simulink model "Monorail_Phase_Shifted_Full_Bridge_Converter"  (R2021b)
settings: Solver=ode1  StartTime=0.0  StopTime=4.00  FixedStep=1e-6  MaxStep=1e-4  RelTol=1e-3  EnableMultiTasking=on
InitFcn:
  | %Input
  | V_supply_max = 910;
  | V_supply_min = 490;
  | R_supply = 1e-06;
  | L_in = 0.5e-03;
  | C_in = 225e-06;
  | 
  | %Control
  | f_sw = 10e03;
  | V_dc_ref = 750;
  | V_dc_init = 450;
  | V_bat_ref = 24;
  | V_bat_init = 14;
  | t_softstart = 0.5;
  | Scale_factor_High = 1/790;
  | Scale_factor_Low = 1/26.26;
  | Kp = 0.5;
  | Ki = pi;
  | PI_max = 0.95;
  | PI_min = 0.05;
  | t_enable = 1e-03;
  | t_dead = 2e-06;
  | 
  | %HF_Transformer
  | P_txf = 50e03;
  | f_txf = 10e03;
  | V_pri_txf = 1e03;
  | V_sec_high_txf = 770;
  | V_sec_low_txf = 27;
  | 
  | %Output
  | L_filt = 1e-03;
  | C_filt = 225e-06;
  | R_load_750V = 750/40;
  | R_load_24V = 24/500;
libraries: spsDiodeLib x12, spsSeriesRLCBranchLib x10, spsIGBTDiodeLib x8, spsCurrentMeasurementLib x3, spsVoltageMeasurementLib x3, simulink x3, spsLinearTransformerLib x2, simulink_extras x2, slpidlib x1, spsControlledVoltageSourceLib x1, spspowerguiLib x1
settings Model: ModifiedByFormat=Sourjya_Mondal  Creator=Sourjya_Mondal  LastModifiedBy=Sourjya_Mondal
settings SolverCC: AlgebraicLoopSolver=TrustRegion
settings DataIOCC: ReturnWorkspaceOutputs=off
settings OptimizationCC: LifeSpan=inf
settings DebuggingCC: SFUnexpectedBacktrackingDiag=warning  SFNoUnconditionalDefaultTransitionDiag=warning  SFExecutionAtInitializationDiag=none  SFMachineParentedDataDiag=warning  ArithmeticOperatorsInVariantConditions=warning
settings SFSimCC: SimUseLocalCustomCode=off  CustomCodeUndefinedFunction=UseInterfaceOnly
settings RTWCC: RTWUseLocalCustomCode=off
settings CodeAppCC: StateflowObjectComments=on
settings GRTTargetCC: TargetLangStandard=C89/C90 (ANSI)
settings ConfigComp: CovMetricSettings=dw  CovSaveCumulativeToWorkspaceVar=on  CovSaveSingleToWorkspaceVar=on  CovExternalEMLEnable=off
settings SimscapeCC: SimscapeNormalizeSystem=off

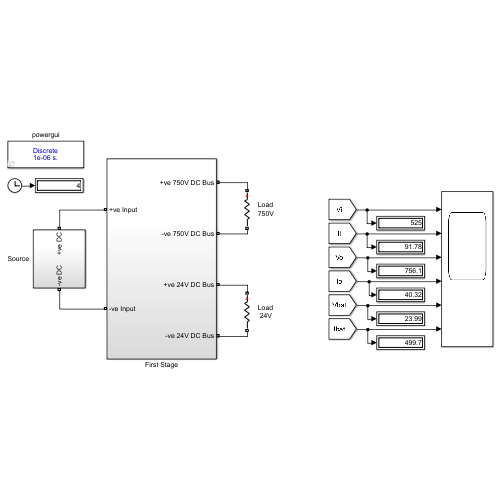
[thumbnail: Simulink's stored preview of the top-level diagram]
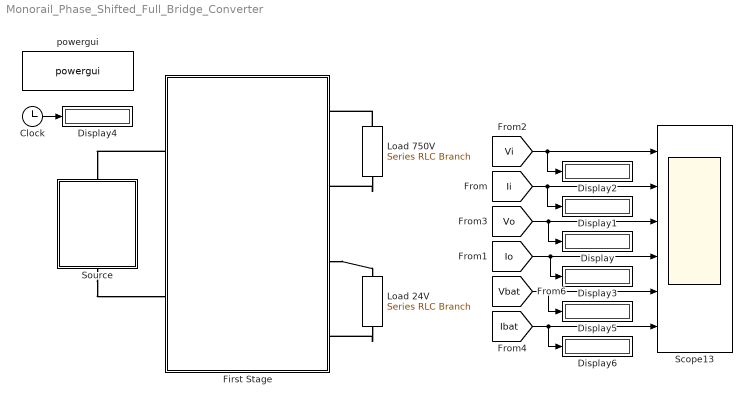
== system Monorail_Phase_Shifted_Full_Bridge_Converter ==
  Clock : Clock
  Display{,1..6} (7 alike) : Display
  First Stage : Subsystem
  Load 24V : spsSeriesRLCBranchLib/Series RLC Branch  LConnTagsString=__new0  RConnTagsString=__new0  BranchType=R  Resistance=R_load_24V  Inductance=1e-3  SetiL0=off  InitialCurrent=0  Capacitance=1e-6  Setx0=off  InitialVoltage=0  Measurements=None
  Load 750V : spsSeriesRLCBranchLib/Series RLC Branch  LConnTagsString=__new0  RConnTagsString=__new0  BranchType=R  Resistance=R_load_750V  Inductance=1e-3  SetiL0=off  InitialCurrent=0  Capacitance=1e-6  Setx0=off  InitialVoltage=0  Measurements=None
  Scope13 : Scope  NumInputPorts=6
  Source : Subsystem
  powergui : spspowerguiLib/powergui  Priority=1  SimulationMode=Discrete  SampleTime=1e-6  frequency=60  Iterations=50  frequencyindice=0  Pbase=100e6  ErrMax=1e-4  UnitsV=kV  UnitsW=MW  buscounter=0  FunctionMessages=off  echomessages=off  EnableUseOfTLC=off  CurrentSourceSwitches=off  DisableSnubberDevices=off  DisableRonSwitches=off  DisableVfSwitches=off  DisplayEquations=off  AutomaticDiscreteSolvers=off  SolverType=Tustin/Backward Euler (TBE)  Interpol=off  ExternalGateDelay=off  methode=off  Ts=100  x0status=blocks  SPID=on  SwTol=0  HookPort=off  NonlinearTolerance=1e-4  nMaxIteration=100  ContinueOnMaxIteration=off  RestoreLinks=warning  ResistiveCurrentMeasurement=off  Frange=[0:2:500]  Ylog=off  Xlog=on  ShowGrid=off  save=off  variable=ZData  structure=ScopeData1  ZoomFFT=on  StartTime=1  cycles=5  DisplayStyle=1  fundamental=50  FreqAxis=off  MaxFrequency=1000  frequencyindicesteady=1  RmsSteady=1  display=off
  wires:
  [Vo] -> Display/1, Scope13/3
  [Io] -> Display3/1, Scope13/4
  [Ii] -> Display1/1, Scope13/2
  [Vi] -> Display2/1, Scope13/1
  Clock/1 -> Display4/1
  [Ibat] -> Scope13/6, Display6/1
  [Vbat] -> Display5/1, Scope13/5
  connections:
  Load 750V/LConn1 -- First Stage/RConn1
  Load 750V/RConn1 -- First Stage/RConn2
  First Stage/RConn3 -- Load 24V/LConn1
  Load 24V/RConn1 -- First Stage/RConn4
  First Stage/LConn1 -- Source/RConn1
  Source/LConn1 -- First Stage/LConn2

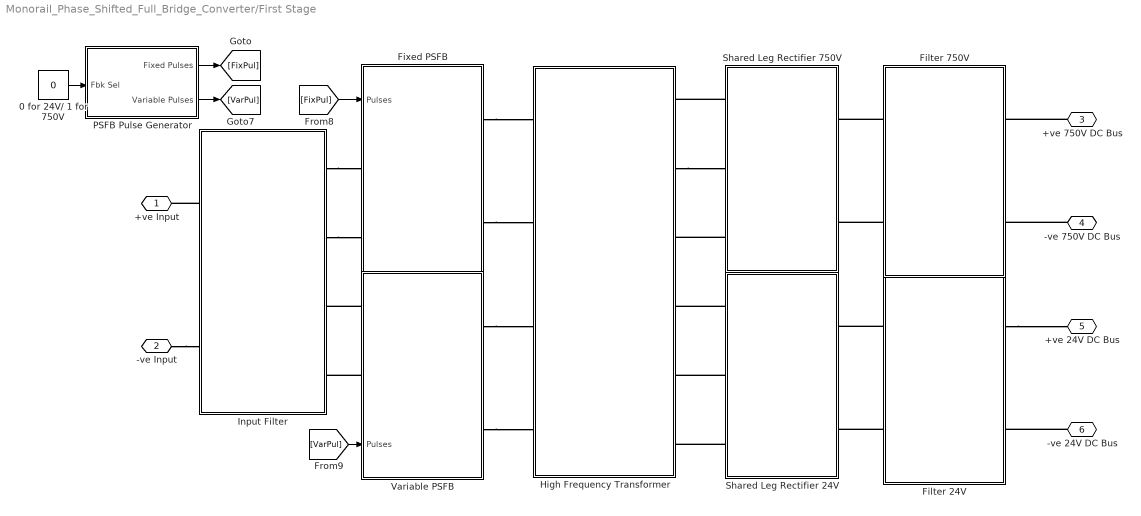
== system Monorail_Phase_Shifted_Full_Bridge_Converter/First Stage ==
  0 for 24V/ 1 for 750V : Constant  Value=0
  Filter 24V : Subsystem
  Filter 750V : Subsystem
  Fixed PSFB : Subsystem
  High Frequency Transformer : Subsystem
  Input Filter : Subsystem
  PSFB Pulse Generator : Subsystem
  Shared Leg Rectifier 24V : Subsystem
  Shared Leg Rectifier 750V : Subsystem
  Variable PSFB : Subsystem
      settings: PortSchema="{\"entries\":[{\"content\":{\"sides\":[{\"content\":{\"connectorIds\":[\"LConn1\",\"LConn2\",\"In1\"]},\"type\":\"ConnectorPlacement.EquallySpacedRectSide\",\"uuid\":\"7757477b-89bb-4ec1-b933-b44ab9d6fde2\"},{\"content\":{\"connectorIds\":[\"RConn1\",\"RConn2\"],\"side\":\"RIGHT\"},\"type\":\"ConnectorPlacement.EquallySpacedRectSide\",\"uuid\":\"8742cb4e-b9ab-4bf3-a691-a84b83766e96\"},{\"content\":{\"connectorIds\":[],\"side\":\"TOP\"},\"type\":\"ConnectorPlacement.EquallySpacedRectSide\",\"uuid\":\"002cf11e-e5e4-407b-9003-66d8e8cf65bf\"}]},\"type\":\"ConnectorPlacement.EquallySpacedConnector\",\"uuid\":\"8388936b-9867-4e43-8ba2-a5a74566d6ba\"}],\"packageUris\":[\"http://schema.mathworks.com/mf0/Connector/19700101\"],\"version\":\"1.0\"}"
  +ve Input : PMIOPort  Side=Left
  -ve Input : PMIOPort  Port=2  Side=Left
  +ve 750V DC Bus : PMIOPort  Port=3  Side=Right
  -ve 750V DC Bus : PMIOPort  Port=4  Side=Right
  +ve 24V DC Bus : PMIOPort  Port=5  Side=Right
  -ve 24V DC Bus : PMIOPort  Port=6  Side=Right
  wires:
  [FixPul] -> Fixed PSFB/1(Pulses)
  0 for 24V/ 1 for 750V/1 -> PSFB Pulse Generator/1(Fbk Sel)
  [VarPul] -> Variable PSFB/1(Pulses)
  PSFB Pulse Generator/2(Variable Pulses) -> [VarPul]
  PSFB Pulse Generator/1(Fixed Pulses) -> [FixPul]
  connections:
  Shared Leg Rectifier 24V/LConn2 -- High Frequency Transformer/RConn5
  Shared Leg Rectifier 24V/LConn1 -- High Frequency Transformer/RConn4
  +ve 750V DC Bus/RConn1 -- Filter 750V/RConn1
  Filter 24V/LConn1 -- Shared Leg Rectifier 24V/RConn1
  Filter 750V/LConn2 -- Shared Leg Rectifier 750V/RConn2
  Filter 24V/LConn2 -- Shared Leg Rectifier 24V/RConn2
  -ve 750V DC Bus/RConn1 -- Filter 750V/RConn2
  Shared Leg Rectifier 24V/LConn3 -- High Frequency Transformer/RConn6
  Fixed PSFB/RConn1 -- High Frequency Transformer/LConn1
  Fixed PSFB/RConn2 -- High Frequency Transformer/LConn2
  High Frequency Transformer/RConn2 -- Shared Leg Rectifier 750V/LConn2
  Shared Leg Rectifier 750V/LConn1 -- High Frequency Transformer/RConn1
  Variable PSFB/RConn1 -- High Frequency Transformer/LConn3
  Shared Leg Rectifier 750V/LConn3 -- High Frequency Transformer/RConn3
  Variable PSFB/RConn2 -- High Frequency Transformer/LConn4
  Filter 750V/LConn1 -- Shared Leg Rectifier 750V/RConn1
  -ve 24V DC Bus/RConn1 -- Filter 24V/RConn2
  Filter 24V/RConn1 -- +ve 24V DC Bus/RConn1
  Input Filter/RConn1 -- Fixed PSFB/LConn1
  Input Filter/RConn2 -- Fixed PSFB/LConn2
  -ve Input/RConn1 -- Input Filter/LConn2
  Variable PSFB/LConn1 -- Input Filter/RConn3
  Variable PSFB/LConn2 -- Input Filter/RConn4
  Input Filter/LConn1 -- +ve Input/RConn1

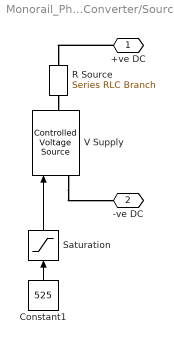
== system Monorail_Phase_Shifted_Full_Bridge_Converter/Source ==
  Constant1 : Constant  Value=525
  R Source : spsSeriesRLCBranchLib/Series RLC Branch  LConnTagsString=__new0  RConnTagsString=__new0  BranchType=R  Resistance=R_supply  Inductance=0.5e-3  SetiL0=off  InitialCurrent=0  Capacitance=1e-6  Setx0=off  InitialVoltage=0  Measurements=None
  Saturation : Saturate  UpperLimit=V_supply_max  LowerLimit=V_supply_min
  V Supply : spsControlledVoltageSourceLib/Controlled Voltage Source  Initialize=on  Source_Type=AC  Amplitude=0  Phase=0  Frequency=0  Measurements=None
  +ve DC : PMIOPort  Side=Right
  -ve DC : PMIOPort  Port=2  Side=Left
  wires:
  Constant1/1 -> Saturation/1
  Saturation/1 -> V Supply/1
  connections:
  +ve DC/RConn1 -- R Source/RConn1
  R Source/LConn1 -- V Supply/RConn1
  V Supply/LConn1 -- -ve DC/RConn1

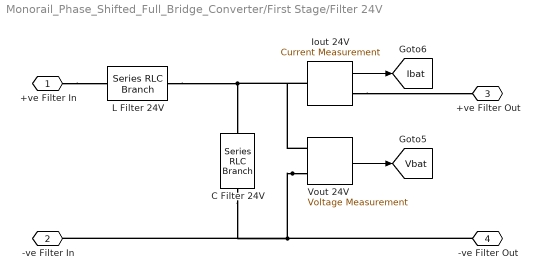
== system Monorail_Phase_Shifted_Full_Bridge_Converter/First Stage/Filter 24V ==
  C Filter 24V : spsSeriesRLCBranchLib/Series RLC Branch  LConnTagsString=__new0  RConnTagsString=__new0  BranchType=C  Resistance=12.25  Inductance=1e-3  SetiL0=off  InitialCurrent=0  Capacitance=C_filt  Setx0=off  InitialVoltage=0  Measurements=None
  Iout 24V : spsCurrentMeasurementLib/Current Measurement  PhasorSimulation=off  OutputType=Complex  PSBequivalent=0
  L Filter 24V : spsSeriesRLCBranchLib/Series RLC Branch  LConnTagsString=__new0  RConnTagsString=__new0  BranchType=L  Resistance=12.25  Inductance=L_filt  SetiL0=off  InitialCurrent=0  Capacitance=1e-6  Setx0=off  InitialVoltage=0  Measurements=None
  Vout 24V : spsVoltageMeasurementLib/Voltage Measurement  PhasorSimulation=off  OutputType=Complex  PSBequivalent=0
  +ve Filter In : PMIOPort  Side=Left
  -ve Filter In : PMIOPort  Port=2  Side=Left
  +ve Filter Out : PMIOPort  Port=3  Side=Right
  -ve Filter Out : PMIOPort  Port=4  Side=Right
  tag scope: Ibat=global, Vbat=global
  wires:
  Vout 24V/1 -> [Vbat]
  Iout 24V/1 -> [Ibat]
  connections:
  Vout 24V/LConn2 -- C Filter 24V/RConn1 -- -ve Filter In/RConn1 -- -ve Filter Out/RConn1
  Iout 24V/RConn1 -- +ve Filter Out/RConn1
  Iout 24V/LConn1 -- Vout 24V/LConn1 -- L Filter 24V/LConn1 -- C Filter 24V/LConn1
  +ve Filter In/RConn1 -- L Filter 24V/RConn1

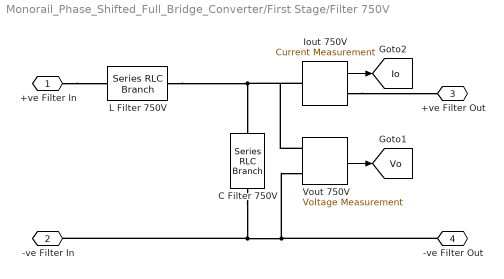
== system Monorail_Phase_Shifted_Full_Bridge_Converter/First Stage/Filter 750V ==
  C Filter 750V : spsSeriesRLCBranchLib/Series RLC Branch  LConnTagsString=__new0  RConnTagsString=__new0  BranchType=C  Resistance=12.25  Inductance=1e-3  SetiL0=off  InitialCurrent=0  Capacitance=C_filt  Setx0=off  InitialVoltage=0  Measurements=None
  Iout 750V : spsCurrentMeasurementLib/Current Measurement  PhasorSimulation=off  OutputType=Complex  PSBequivalent=0
  L Filter 750V : spsSeriesRLCBranchLib/Series RLC Branch  LConnTagsString=__new0  RConnTagsString=__new0  BranchType=L  Resistance=12.25  Inductance=L_filt  SetiL0=off  InitialCurrent=0  Capacitance=1e-6  Setx0=off  InitialVoltage=0  Measurements=None
  Vout 750V : spsVoltageMeasurementLib/Voltage Measurement  PhasorSimulation=off  OutputType=Complex  PSBequivalent=0
  +ve Filter In : PMIOPort  Side=Left
  -ve Filter In : PMIOPort  Port=2  Side=Left
  +ve Filter Out : PMIOPort  Port=3  Side=Right
  -ve Filter Out : PMIOPort  Port=4  Side=Right
  tag scope: Io=global, Vo=global
  wires:
  Vout 750V/1 -> [Vo]
  Iout 750V/1 -> [Io]
  connections:
  +ve Filter In/RConn1 -- L Filter 750V/RConn1
  L Filter 750V/LConn1 -- Iout 750V/LConn1 -- Vout 750V/LConn1 -- C Filter 750V/LConn1
  Iout 750V/RConn1 -- +ve Filter Out/RConn1
  C Filter 750V/RConn1 -- Vout 750V/LConn2 -- -ve Filter Out/RConn1 -- -ve Filter In/RConn1

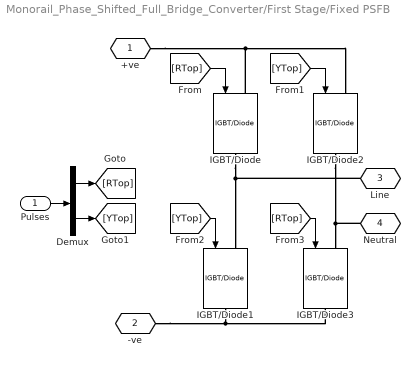
== system Monorail_Phase_Shifted_Full_Bridge_Converter/First Stage/Fixed PSFB ==
  Pulses : Inport
  Demux : Demux  Outputs=2
  IGBT/Diode{,1..3} (4 alike) : spsIGBTDiodeLib/IGBT//Diode  Ron=1e-3  Rs=1e5  Cs=inf  Measurements=off
  +ve : PMIOPort  Side=Left
  -ve : PMIOPort  Port=2  Side=Left
  Line : PMIOPort  Port=3  Side=Right
  Neutral : PMIOPort  Port=4  Side=Right
  wires:
  [RTop] -> IGBT/Diode/1
  [RTop] -> IGBT/Diode3/1
  [YTop] -> IGBT/Diode1/1
  [YTop] -> IGBT/Diode2/1
  Demux/1 -> [RTop]
  Demux/2 -> [YTop]
  Pulses/1 -> Demux/1
  connections:
  IGBT/Diode2/RConn1 -- IGBT/Diode3/LConn1 -- Neutral/RConn1
  IGBT/Diode/RConn1 -- Line/RConn1 -- IGBT/Diode1/LConn1
  IGBT/Diode/LConn1 -- +ve/RConn1 -- IGBT/Diode2/LConn1
  IGBT/Diode1/RConn1 -- IGBT/Diode3/RConn1 -- -ve/RConn1

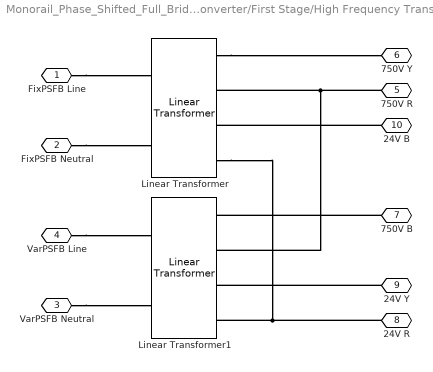
== system Monorail_Phase_Shifted_Full_Bridge_Converter/First Stage/High Frequency Transformer ==
  Linear Transformer : spsLinearTransformerLib/Linear Transformer  UNITS=SI  NominalPower=[P_txf f_txf]  winding1=[V_pri_txf 0 0]  winding2=[V_sec_high_txf 0 0]  ThreeWindings=on  winding3=[V_sec_low_txf 0 0]  RmLm=[inf inf]  Measurements=None  DataType=on
  Linear Transformer1 : spsLinearTransformerLib/Linear Transformer  UNITS=SI  NominalPower=[P_txf f_txf]  winding1=[V_pri_txf 0 0]  winding2=[V_sec_high_txf 0 0]  ThreeWindings=on  winding3=[V_sec_low_txf 0 0]  RmLm=[inf inf]  Measurements=None  DataType=on
  FixPSFB Line : PMIOPort  Side=Left
  FixPSFB Neutral : PMIOPort  Port=2  Side=Left
  VarPSFB Neutral : PMIOPort  Port=3  Side=Left
  VarPSFB Line : PMIOPort  Port=4  Side=Left
  750V R : PMIOPort  Port=5  Side=Right
  750V Y : PMIOPort  Port=6  Side=Right
  750V B : PMIOPort  Port=7  Side=Right
  24V R : PMIOPort  Port=8  Side=Right
  24V Y : PMIOPort  Port=9  Side=Right
  24V B : PMIOPort  Port=10  Side=Right
  connections:
  FixPSFB Line/RConn1 -- Linear Transformer/LConn1
  Linear Transformer/RConn1 -- 750V Y/RConn1
  Linear Transformer/RConn4 -- Linear Transformer1/RConn4 -- 24V R/RConn1
  750V R/RConn1 -- Linear Transformer/RConn2 -- Linear Transformer1/RConn2
  24V Y/RConn1 -- Linear Transformer1/RConn3
  VarPSFB Neutral/RConn1 -- Linear Transformer1/LConn2
  750V B/RConn1 -- Linear Transformer1/RConn1
  VarPSFB Line/RConn1 -- Linear Transformer1/LConn1
  FixPSFB Neutral/RConn1 -- Linear Transformer/LConn2
  24V B/RConn1 -- Linear Transformer/RConn3

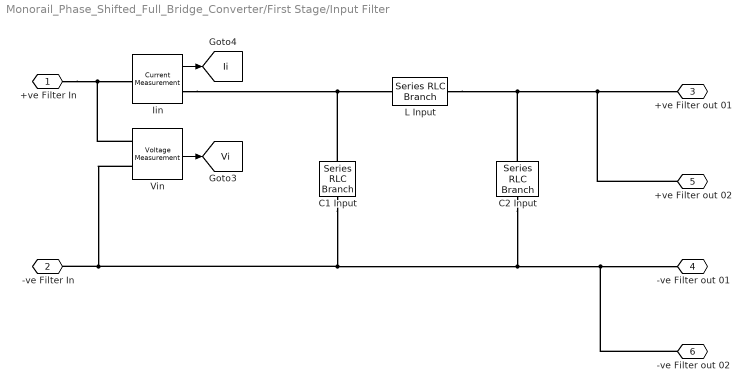
== system Monorail_Phase_Shifted_Full_Bridge_Converter/First Stage/Input Filter ==
  C1 Input : spsSeriesRLCBranchLib/Series RLC Branch  LConnTagsString=__new0  RConnTagsString=__new0  BranchType=C  Resistance=0.1  Inductance=1e-3  SetiL0=off  InitialCurrent=0  Capacitance=C_in  Setx0=off  InitialVoltage=0  Measurements=None
  C2 Input : spsSeriesRLCBranchLib/Series RLC Branch  LConnTagsString=__new0  RConnTagsString=__new0  BranchType=C  Resistance=12.25  Inductance=1e-3  SetiL0=off  InitialCurrent=0  Capacitance=C_in  Setx0=off  InitialVoltage=0  Measurements=None
  Iin : spsCurrentMeasurementLib/Current Measurement  PhasorSimulation=off  OutputType=Complex  PSBequivalent=0
  L Input : spsSeriesRLCBranchLib/Series RLC Branch  LConnTagsString=__new0  RConnTagsString=__new0  BranchType=L  Resistance=12.25  Inductance=L_in  SetiL0=off  InitialCurrent=0  Capacitance=1e-6  Setx0=off  InitialVoltage=0  Measurements=None
  Vin : spsVoltageMeasurementLib/Voltage Measurement  PhasorSimulation=off  OutputType=Complex  PSBequivalent=0
  +ve Filter In : PMIOPort  Side=Left
  -ve Filter In : PMIOPort  Port=2  Side=Left
  +ve Filter out 01 : PMIOPort  Port=3  Side=Right
  -ve Filter out 01 : PMIOPort  Port=4  Side=Right
  +ve Filter out 02 : PMIOPort  Port=5  Side=Right
  -ve Filter out 02 : PMIOPort  Port=6  Side=Right
  tag scope: Ii=global, Vi=global
  wires:
  Vin/1 -> [Vi]
  Iin/1 -> [Ii]
  connections:
  C1 Input/LConn1 -- Iin/RConn1 -- L Input/LConn1
  C1 Input/RConn1 -- C2 Input/RConn1 -- -ve Filter out 02/RConn1 -- -ve Filter out 01/RConn1 -- Vin/LConn2 -- -ve Filter In/RConn1
  L Input/RConn1 -- C2 Input/LConn1 -- +ve Filter out 02/RConn1 -- +ve Filter out 01/RConn1
  Vin/LConn1 -- +ve Filter In/RConn1 -- Iin/LConn1

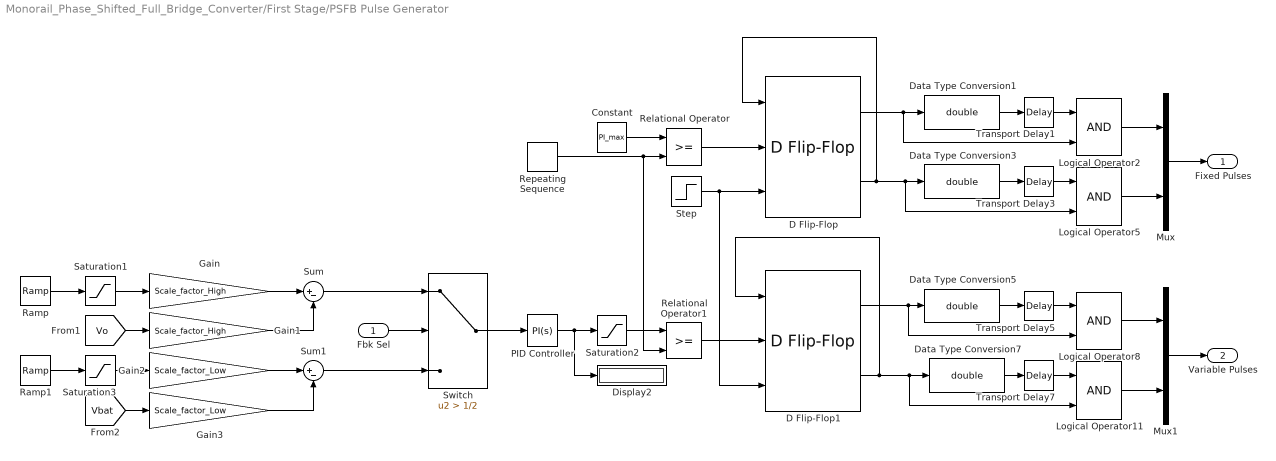
== system Monorail_Phase_Shifted_Full_Bridge_Converter/First Stage/PSFB Pulse Generator ==
  Fbk Sel : Inport
  Constant : Constant  Value=PI_max
  D Flip-Flop : simulink_extras/Flip Flops/D Flip-Flop
  D Flip-Flop1 : simulink_extras/Flip Flops/D Flip-Flop
  Data Type Conversion{1,3,5,7} (4 alike) : DataTypeConversion  OutDataTypeStr=double
  Display2 : Display
  Gain : Gain  Gain=Scale_factor_High
  Gain1 : Gain  Gain=Scale_factor_High
  Gain2 : Gain  Gain=Scale_factor_Low
  Gain3 : Gain  Gain=Scale_factor_Low
  Logical Operator{2,5,8,11} (4 alike) : Logic  IconShape=distinctive  AllPortsSameDT=off  OutDataTypeStr=boolean
  Mux : Mux  Inputs=2
  Mux1 : Mux  Inputs=2
  PID Controller : slpidlib/PID Controller  Controller=PI  Form=Parallel  TimeDomain=Continuous-time  UseExternalTs=off  SampleTime=-1  IntegratorMethod=Forward Euler  FilterMethod=Forward Euler  ControllerParametersSource=internal  P=Kp  I=Ki  D=0  UseFilter=on  N=100  TunerSelectOption=Transfer Function Based (PID Tuner App)  InitialConditionSource=internal  InitialConditionForIntegrator=0  InitialConditionForFilter=0  DifferentiatorICPrevScaledInput=0  ExternalReset=none  TrackingMode=off  Kt=1  LimitOutput=off  SatLimitsSource=internal  UpperSaturationLimit=inf  LowerSaturationLimit=-inf  LinearizeAsGain=on  AntiWindupMode=none  Kb=1  POutMin=[]  POutMax=[]  IOutMin=[]  IOutMax=[]  DOutMin=[]  DOutMax=[]  NOutMin=[]  NOutMax=[]  SumOutMin=[]  SumOutMax=[]  SaturationOutMin=[]  SaturationOutMax=[]  PParamMin=[]  PParamMax=[]  IParamMin=[]  IParamMax=[]  DParamMin=[]  DParamMax=[]  NParamMin=[]  NParamMax=[]  KbParamMin=[]  KbParamMax=[]  KtParamMin=[]  KtParamMax=[]  KbOutMin=[]  KbOutMax=[]  KtOutMin=[]  KtOutMax=[]  IntegratorOutMin=[]  IntegratorOutMax=[]  FilterOutMin=[]  FilterOutMax=[]  SumI1OutMin=[]  SumI1OutMax=[]  SumI2OutMin=[]  SumI2OutMax=[]  SumI3OutMin=[]  SumI3OutMax=[]  SumI4OutMin=[]  SumI4OutMax=[]  SumDOutMin=[]  SumDOutMax=[]  DifferentiatorOutMin=[]  DifferentiatorOutMax=[]  FilterDiffOutCoefMin=[]  FilterDiffOutCoefMax=[]  ReciprocalOutMin=[]  ReciprocalOutMax=[]  SumDenOutMin=[]  SumDenOutMax=[]  SumNumOutMin=[]  SumNumOutMax=[]  DivideOutMin=[]  DivideOutMax=[]  UdiffTsProdOutMin=[]  UdiffTsProdOutMax=[]  NTsProdOutMin=[]  NTsProdOutMax=[]  UintegralTsProdOutMin=[]  UintegralTsProdOutMax=[]  UngainTsProdOutMin=[]  UngainTsProdOutMax=[]  IntegratorContinuousStateAttributes=''  IntegratorStateMustResolveToSignalObject=off  IntegratorRTWStateStorageClass=Auto  FilterContinuousStateAttributes=''  FilterStateMustResolveToSignalObject=off  FilterRTWStateStorageClass=Auto  ParallelPVariant=InternalParameters  IdealPVariant=Disabled  IVariant=InternalParameters  DVariant=Disabled  IntegratorVariant=Continuous  SatVariant=Disabled  AWVariant=Passthrough  PCopyVariant=Disabled  TRVariant=Disabled  FdbkBlocksVariant=Forward  IdealPFdbkVariant=Disabled  SatFdbkVariant=Disabled  DerivativeFilterVariant=Disabled  NVariant=Disabled  NCopyVariant=Disabled_SignalSpec  FilterICVariant=Disabled  IntegratorICVariant=InternalICs  ExternalResetVariant=Disabled  TRSumVariant=Passthrough  SumFdbkVariant=Disabled  SumVariant=Sum_PI  TsampFilterVariant=InternalTs  TsampNgainVariant=Passthrough  TsampIntegralVariant=Passthrough  ExternalSaturationOutDataTypeStr=Inherit: Same as second input
  Ramp : simulink/Sources/Ramp  slope=V_dc_ref/t_softstart  start=0  InitialOutput=0
  Ramp1 : simulink/Sources/Ramp  slope=V_bat_ref/t_softstart  start=0  InitialOutput=0
  Relational Operator : RelationalOperator  OutDataTypeStr=boolean  RndMeth=Nearest
  Relational Operator1 : RelationalOperator  OutDataTypeStr=boolean  RndMeth=Nearest
  Repeating Sequence : simulink/Sources/Repeating Sequence  rep_seq_t=[0 1/(2*f_sw)]  rep_seq_y=[1 0]
  Saturation1 : Saturate  UpperLimit=V_dc_ref  LowerLimit=V_dc_init  ZeroCross=off
  Saturation2 : Saturate  UpperLimit=PI_max  LowerLimit=PI_min  ZeroCross=off
  Saturation3 : Saturate  UpperLimit=V_bat_ref  LowerLimit=V_bat_init  ZeroCross=off
  Step : Step  Time=t_enable  SampleTime=0
  Sum : Sum  Inputs=|+-
  Sum1 : Sum  Inputs=|+-
  Switch : Switch  Criteria=u2 > Threshold  Threshold=1/2
  Transport Delay{1,3,5,7} (4 alike) : TransportDelay  DelayTime=t_dead
  Fixed Pulses : Outport
  Variable Pulses : Outport  Port=2
  wires:
  Data Type Conversion7/1 -> Transport Delay7/1
  Constant/1 -> Relational Operator/1
  D Flip-Flop/1 -> Logical Operator2/2, Data Type Conversion1/1
  Relational Operator1/1 -> D Flip-Flop1/2
  D Flip-Flop1/1 -> Logical Operator8/2, Data Type Conversion5/1
  D Flip-Flop/2 -> Logical Operator5/2, Data Type Conversion3/1, D Flip-Flop/1
  D Flip-Flop1/2 -> Logical Operator11/2, Data Type Conversion7/1, D Flip-Flop1/1
  Data Type Conversion5/1 -> Transport Delay5/1
  Step/1 -> D Flip-Flop/3, D Flip-Flop1/3
  Relational Operator/1 -> D Flip-Flop/2
  Data Type Conversion1/1 -> Transport Delay1/1
  Transport Delay1/1 -> Logical Operator2/1
  [Vo] -> Gain1/1
  Transport Delay7/1 -> Logical Operator11/1
  Repeating Sequence/1 -> Relational Operator/2, Relational Operator1/2
  Saturation2/1 -> Relational Operator1/1
  Logical Operator8/1 -> Mux1/1
  Logical Operator2/1 -> Mux/1
  Saturation1/1 -> Gain/1
  Logical Operator5/1 -> Mux/2
  Ramp/1 -> Saturation1/1
  Data Type Conversion3/1 -> Transport Delay3/1
  Transport Delay3/1 -> Logical Operator5/1
  Transport Delay5/1 -> Logical Operator8/1
  Logical Operator11/1 -> Mux1/2
  Mux/1 -> Fixed Pulses/1
  Mux1/1 -> Variable Pulses/1
  Gain/1 -> Sum/1
  Gain1/1 -> Sum/2
  Gain3/1 -> Sum1/2
  Gain2/1 -> Sum1/1
  Ramp1/1 -> Saturation3/1
  Saturation3/1 -> Gain2/1
  [Vbat] -> Gain3/1
  Fbk Sel/1 -> Switch/2
  Switch/1 -> PID Controller/1
  Sum/1 -> Switch/1
  Sum1/1 -> Switch/3
  PID Controller/1 -> Display2/1, Saturation2/1

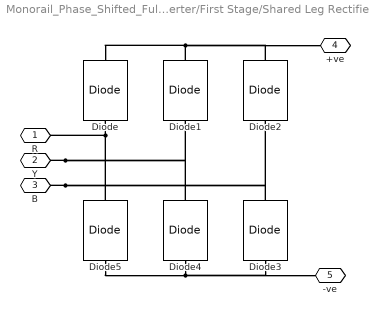
== system Monorail_Phase_Shifted_Full_Bridge_Converter/First Stage/Shared Leg Rectifier 24V ==
  Diode{,1..5} (6 alike) : spsDiodeLib/Diode  Ron=0.001  Lon=0  Vf=0.8  IC=0  UseSnubber=0  Rs=500  Cs=250e-9  Measurements=off
  R : PMIOPort  Side=Left
  Y : PMIOPort  Port=2  Side=Left
  B : PMIOPort  Port=3  Side=Left
  +ve : PMIOPort  Port=4  Side=Right
  -ve : PMIOPort  Port=5  Side=Right
  connections:
  Diode/LConn1 -- R/RConn1 -- Diode5/RConn1
  Diode4/LConn1 -- -ve/RConn1 -- Diode3/LConn1 -- Diode5/LConn1
  B/RConn1 -- Diode2/LConn1 -- Diode3/RConn1
  Diode1/RConn1 -- Diode2/RConn1 -- +ve/RConn1 -- Diode/RConn1
  Y/RConn1 -- Diode1/LConn1 -- Diode4/RConn1

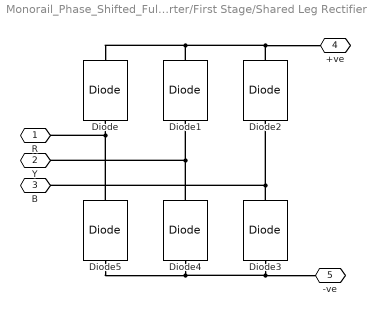
== system Monorail_Phase_Shifted_Full_Bridge_Converter/First Stage/Shared Leg Rectifier 750V ==
  Diode{,1..5} (6 alike) : spsDiodeLib/Diode  Ron=0.001  Lon=0  Vf=0.8  IC=0  UseSnubber=0  Rs=500  Cs=250e-9  Measurements=off
  R : PMIOPort  Side=Left
  Y : PMIOPort  Port=2  Side=Left
  B : PMIOPort  Port=3  Side=Left
  +ve : PMIOPort  Port=4  Side=Right
  -ve : PMIOPort  Port=5  Side=Right
  connections:
  Diode4/RConn1 -- Diode1/LConn1 -- Y/RConn1
  Diode/RConn1 -- +ve/RConn1 -- Diode2/RConn1 -- Diode1/RConn1
  Diode3/RConn1 -- Diode2/LConn1 -- B/RConn1
  Diode5/LConn1 -- Diode3/LConn1 -- -ve/RConn1 -- Diode4/LConn1
  Diode5/RConn1 -- R/RConn1 -- Diode/LConn1

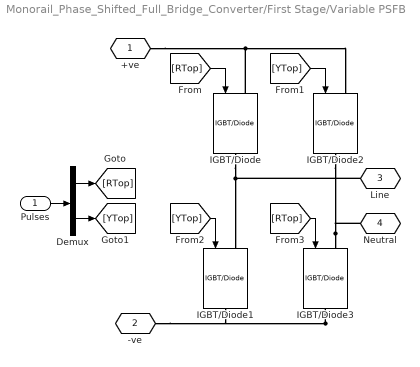
== system Monorail_Phase_Shifted_Full_Bridge_Converter/First Stage/Variable PSFB ==
  Pulses : Inport
  Demux : Demux  Outputs=2
  IGBT/Diode{,1..3} (4 alike) : spsIGBTDiodeLib/IGBT//Diode  Ron=1e-3  Rs=1e5  Cs=inf  Measurements=off
  +ve : PMIOPort  Side=Left
  -ve : PMIOPort  Port=2  Side=Left
  Line : PMIOPort  Port=3  Side=Right
  Neutral : PMIOPort  Port=4  Side=Right
  wires:
  Pulses/1 -> Demux/1
  Demux/2 -> [YTop]
  Demux/1 -> [RTop]
  [YTop] -> IGBT/Diode2/1
  [YTop] -> IGBT/Diode1/1
  [RTop] -> IGBT/Diode3/1
  [RTop] -> IGBT/Diode/1
  connections:
  IGBT/Diode3/RConn1 -- -ve/RConn1 -- IGBT/Diode1/RConn1
  +ve/RConn1 -- IGBT/Diode/LConn1 -- IGBT/Diode2/LConn1
  Line/RConn1 -- IGBT/Diode1/LConn1 -- IGBT/Diode/RConn1
  IGBT/Diode3/LConn1 -- Neutral/RConn1 -- IGBT/Diode2/RConn1
